simulink model "untitled1"  (R2022a)
settings: Solver=VariableStepAuto  StartTime=0.0  StopTime=2  MaxStep=0.005  RelTol=1e-3
values from neighbouring files (symbols this model uses):
  D_1 = 0.0001    [WS.m]
  D_2 = 0.0001    [WS.m]
  E_1 = 8.25 * 10^4    (= 82500)    [WS.m]
  E_2 = 8.25 * 10^4    (= 82500)    [WS.m]
  gy = 0    [WS.m]
  gz = 0    [WS.m]
  Imx_1 = 1.0053e-07    [WS.m]
  Imx_2 = 1.0053e-07    [WS.m]
  Ix_1 = 10^-5    (= 1e-05)    [WS.m]
  Ix_2 = 10^-5    (= 1e-05)    [WS.m]
  k_1_0 = 0.1    [WS.m]
  k_2_0 = 0.1    [WS.m]
  k_dot_1_0 = 0    [WS.m]
  k_dot_2_0 = 0    [WS.m]
  l_1 = 0.05    [WS.m]
  l_2 = 0.05    [WS.m]
  m_1 = 0.08    [WS.m]
  m_2 = 0.08    [WS.m]
  p_tendon_0 = [0.012,0,0]    [WS.m]
  p_tendon_1 = [0.012,0,0]    [WS.m]
  p_tendon_2 = [0.012,0,0]    [WS.m]
libraries: slpidlib x1, matrix_library x1
settings Model: Creator=luca  LastModifiedBy=atled
settings SolverCC: MaxConsecutiveMinStep=20

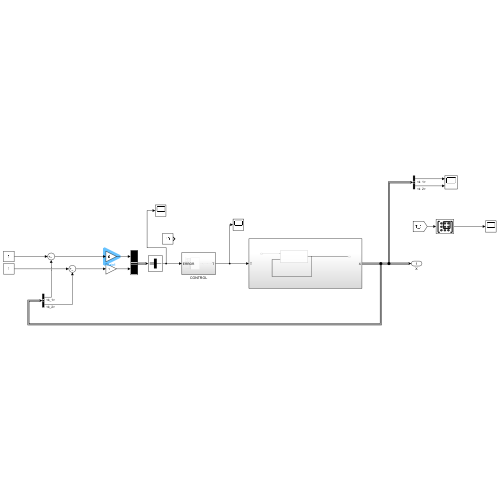
[thumbnail: Simulink's stored preview of the top-level diagram]
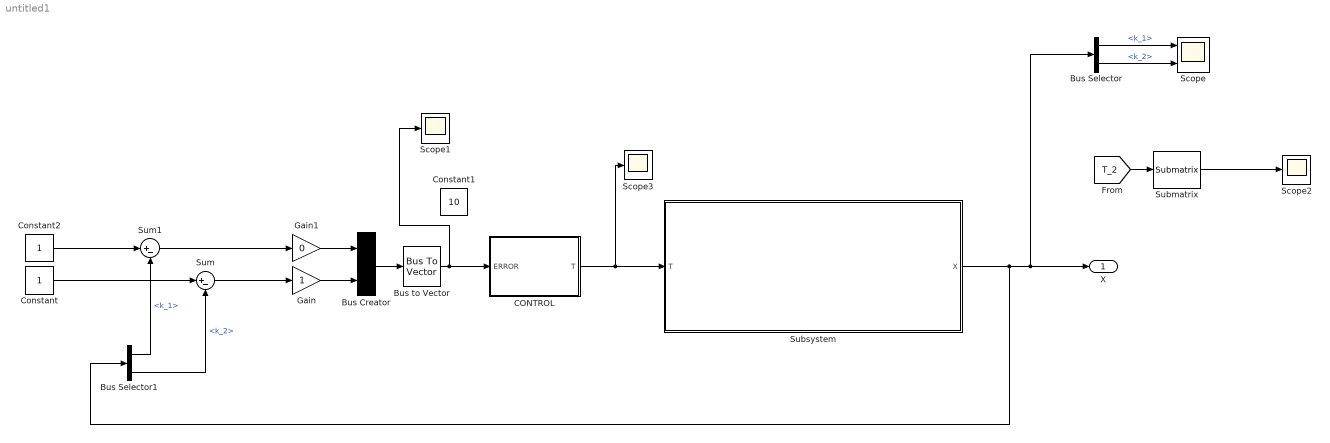
== system untitled1 ==
  Bus Creator : BusCreator  Inputs=2
  Bus Selector : BusSelector  OutputSignals=q.k_1,q.k_2
  Bus Selector1 : BusSelector  OutputSignals=q.k_1,q.k_2
  Bus to Vector : BusToVector
  CONTROL : Subsystem
  Constant : Constant  VectorParams1D=off
  Constant1 : Constant  Value=10  VectorParams1D=off
  Constant2 : Constant  VectorParams1D=off
  Gain : Gain
  Gain1 : Gain  Gain=0
  Scope : Scope  NumInputPorts=2
  Scope1 : Scope
  Scope2 : Scope
  Scope3 : Scope
  Submatrix : matrix_library/Submatrix  RowSpan=Range of rows  RowStartMode=Index  RowStartIndex=1  RowEndMode=Index  RowEndIndex=3  ColSpan=One column  ColStartMode=Last  ColStartIndex=1  ColEndMode=Last  ColEndIndex=1
      settings: SourceProductBaseCode=SL
  Subsystem : Subsystem
  Sum : Sum  Inputs=|+-
  Sum1 : Sum  Inputs=|+-
  X : Outport
  wires:
  Subsystem/1(X) -> Bus Selector1/1, Bus Selector/1, X/1
  Bus Selector/1 -> Scope/1  "<k_1>"
  Bus Selector/2 -> Scope/2  "<k_2>"
  Constant/1 -> Sum/1
  [T_2] -> Submatrix/1
  Submatrix/1 -> Scope2/1
  Sum/1 -> Gain/1
  Constant2/1 -> Sum1/1
  Bus Selector1/1 -> Sum1/2  "<k_1>"
  Bus Selector1/2 -> Sum/2  "<k_2>"
  Sum1/1 -> Gain1/1
  Bus to Vector/1 -> Scope1/1, CONTROL/1(ERROR)
  Gain1/1 -> Bus Creator/1
  Gain/1 -> Bus Creator/2
  CONTROL/1(T) -> Scope3/1, Subsystem/1(T)
  Bus Creator/1 -> Bus to Vector/1

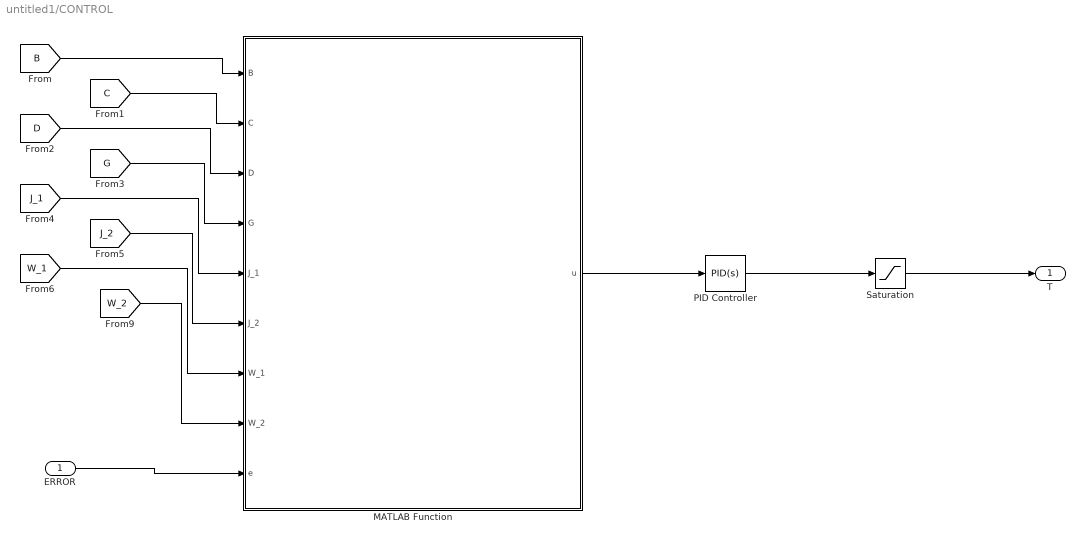
== system untitled1/CONTROL ==
  ERROR : Inport
  MATLAB Function : MATLAB Function  TreatAsAtomicUnit=on
  PID Controller : slpidlib/PID Controller  Controller=PID  Form=Parallel  TimeDomain=Continuous-time  UseExternalTs=off  SampleTime=-1  IntegratorMethod=Forward Euler  FilterMethod=Forward Euler  ControllerParametersSource=internal  P=-3  I=0  UseKiTs=off  D=0.02  N=100  UseFilter=on  TunerSelectOption=Transfer Function Based (PID Tuner App)  InitialConditionSource=internal  InitialConditionForIntegrator=0  InitialConditionForFilter=0  DifferentiatorICPrevScaledInput=0  ExternalReset=none  TrackingMode=off  Kt=1  LimitOutput=off  SatLimitsSource=internal  UpperSaturationLimit=inf  LowerSaturationLimit=-inf  LinearizeAsGain=on  AntiWindupMode=none  Kb=1  POutMin=[]  POutMax=[]  IOutMin=[]  IOutMax=[]  DOutMin=[]  DOutMax=[]  NOutMin=[]  NOutMax=[]  SumOutMin=[]  SumOutMax=[]  SaturationOutMin=[]  SaturationOutMax=[]  PParamMin=[]  PParamMax=[]  IParamMin=[]  IParamMax=[]  DParamMin=[]  DParamMax=[]  NParamMin=[]  NParamMax=[]  KbParamMin=[]  KbParamMax=[]  KtParamMin=[]  KtParamMax=[]  KbOutMin=[]  KbOutMax=[]  KtOutMin=[]  KtOutMax=[]  IntegratorOutMin=[]  IntegratorOutMax=[]  FilterOutMin=[]  FilterOutMax=[]  SumI1OutMin=[]  SumI1OutMax=[]  SumI2OutMin=[]  SumI2OutMax=[]  SumI3OutMin=[]  SumI3OutMax=[]  SumI4OutMin=[]  SumI4OutMax=[]  SumDOutMin=[]  SumDOutMax=[]  DifferentiatorOutMin=[]  DifferentiatorOutMax=[]  FilterDiffOutCoefMin=[]  FilterDiffOutCoefMax=[]  ReciprocalOutMin=[]  ReciprocalOutMax=[]  SumDenOutMin=[]  SumDenOutMax=[]  SumNumOutMin=[]  SumNumOutMax=[]  DivideOutMin=[]  DivideOutMax=[]  UdiffTsProdOutMin=[]  UdiffTsProdOutMax=[]  NTsProdOutMin=[]  NTsProdOutMax=[]  UintegralTsProdOutMin=[]  UintegralTsProdOutMax=[]  UngainTsProdOutMin=[]  UngainTsProdOutMax=[]  IntegratorContinuousStateAttributes=''  IntegratorStateMustResolveToSignalObject=off  IntegratorRTWStateStorageClass=Auto  FilterContinuousStateAttributes=''  FilterStateMustResolveToSignalObject=off  FilterRTWStateStorageClass=Auto  ParallelPVariant=InternalParameters  IdealPVariant=Disabled  IVariant=InternalParameters  DVariant=InternalParameters  IntegratorVariant=Continuous  SatVariant=Disabled  AWVariant=Passthrough  PCopyVariant=Disabled  TRVariant=Disabled  FdbkBlocksVariant=Forward  IdealPFdbkVariant=Disabled  SatFdbkVariant=Disabled  DerivativeFilterVariant=ContFilter  NVariant=InternalParameters  NCopyVariant=Disabled  FilterICVariant=InternalICsFilter  IntegratorICVariant=InternalICs  ExternalResetVariant=Disabled  TRSumVariant=Passthrough  SumFdbkVariant=Disabled  SumVariant=Sum_PID  TsampFilterVariant=InternalTs  TsampNgainVariant=Passthrough  TsampIntegralVariant=Passthrough  ExternalSaturationOutDataTypeStr=Inherit: Same as second input  aMode=0
  Saturation : Saturate  UpperLimit=50  LowerLimit=0
  T : Outport
  wires:
  [B] -> MATLAB Function/1(B)
  [C] -> MATLAB Function/2(C)
  [J_1] -> MATLAB Function/5(J_1)
  [G] -> MATLAB Function/4(G)
  [W_2] -> MATLAB Function/8(W_2)
  [J_2] -> MATLAB Function/6(J_2)
  [D] -> MATLAB Function/3(D)
  [W_1] -> MATLAB Function/7(W_1)
  ERROR/1 -> MATLAB Function/9(e)
  PID Controller/1 -> Saturation/1
  MATLAB Function/1(u) -> PID Controller/1
  Saturation/1 -> T/1

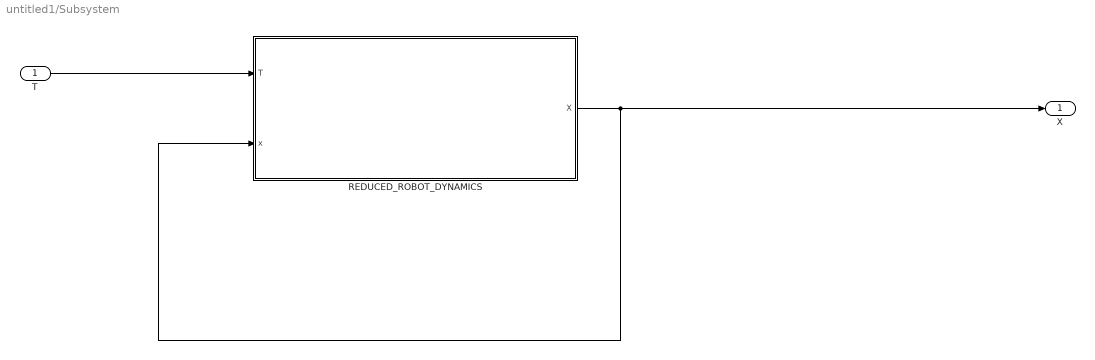
== system untitled1/Subsystem ==
  T : Inport
  REDUCED_ROBOT_DYNAMICS : Subsystem
  X : Outport
  wires:
  T/1 -> REDUCED_ROBOT_DYNAMICS/1(T)
  REDUCED_ROBOT_DYNAMICS/1(X) -> X/1, REDUCED_ROBOT_DYNAMICS/2(x)

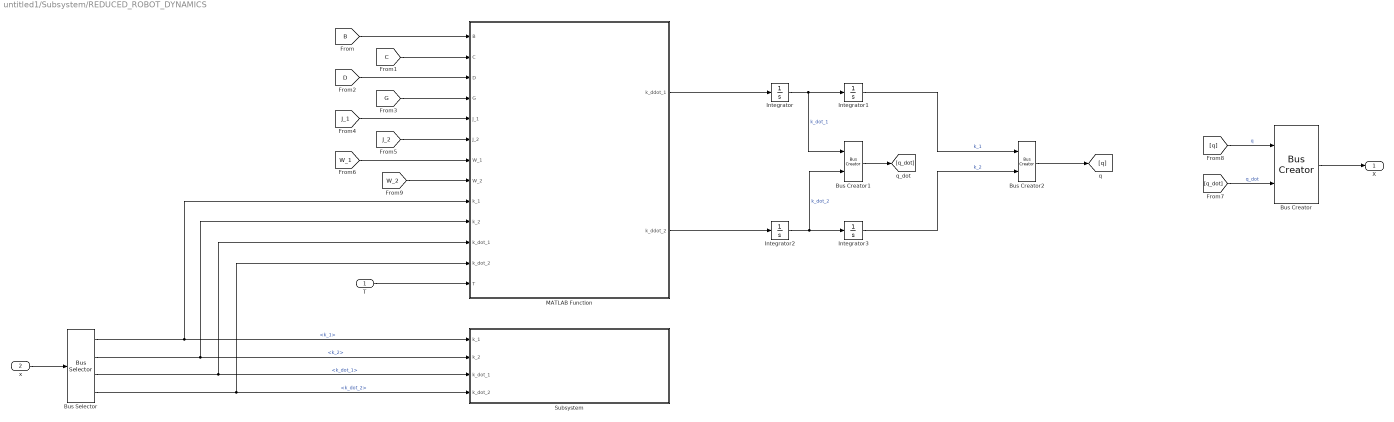
== system untitled1/Subsystem/REDUCED_ROBOT_DYNAMICS ==
  T : Inport
  x : Inport  Port=2
  Bus Creator : BusCreator  Inputs=2
  Bus Creator1 : BusCreator  Inputs=2
  Bus Creator2 : BusCreator  Inputs=2
  Bus Selector : BusSelector  OutputSignals=q.k_1,q.k_2,q_dot.k_dot_1,q_dot.k_dot_2
  Integrator : Integrator  InitialCondition=k_dot_1_0
  Integrator1 : Integrator  InitialCondition=k_1_0
  Integrator2 : Integrator  InitialCondition=k_dot_2_0
  Integrator3 : Integrator  InitialCondition=k_2_0
  MATLAB Function : MATLAB Function  TreatAsAtomicUnit=on
  Subsystem : Subsystem
  X : Outport
  wires:
  T/1 -> MATLAB Function/13(T)
  Bus Creator/1 -> X/1
  Bus Selector/1 -> MATLAB Function/9(k_1), Subsystem/1(k_1)  "<k_1>"
  Integrator2/1 -> Bus Creator1/2, Integrator3/1  "k_dot_2"
  [q] -> Bus Creator/1  "q"
  [q_dot] -> Bus Creator/2  "q_dot"
  [B] -> MATLAB Function/1(B)
  [W_1] -> MATLAB Function/7(W_1)
  [J_2] -> MATLAB Function/6(J_2)
  x/1 -> Bus Selector/1
  Integrator/1 -> Bus Creator1/1, Integrator1/1  "k_dot_1"
  [C] -> MATLAB Function/2(C)
  Bus Creator2/1 -> [q]
  Integrator3/1 -> Bus Creator2/2  "k_2"
  MATLAB Function/1(k_ddot_1) -> Integrator/1
  Bus Creator1/1 -> [q_dot]
  [D] -> MATLAB Function/3(D)
  MATLAB Function/2(k_ddot_2) -> Integrator2/1
  Bus Selector/4 -> MATLAB Function/12(k_dot_2), Subsystem/4(k_dot_2)  "<k_dot_2>"
  Bus Selector/3 -> MATLAB Function/11(k_dot_1), Subsystem/3(k_dot_1)  "<k_dot_1>"
  Integrator1/1 -> Bus Creator2/1  "k_1"
  [J_1] -> MATLAB Function/5(J_1)
  Bus Selector/2 -> MATLAB Function/10(k_2), Subsystem/2(k_2)  "<k_2>"
  [G] -> MATLAB Function/4(G)
  [W_2] -> MATLAB Function/8(W_2)

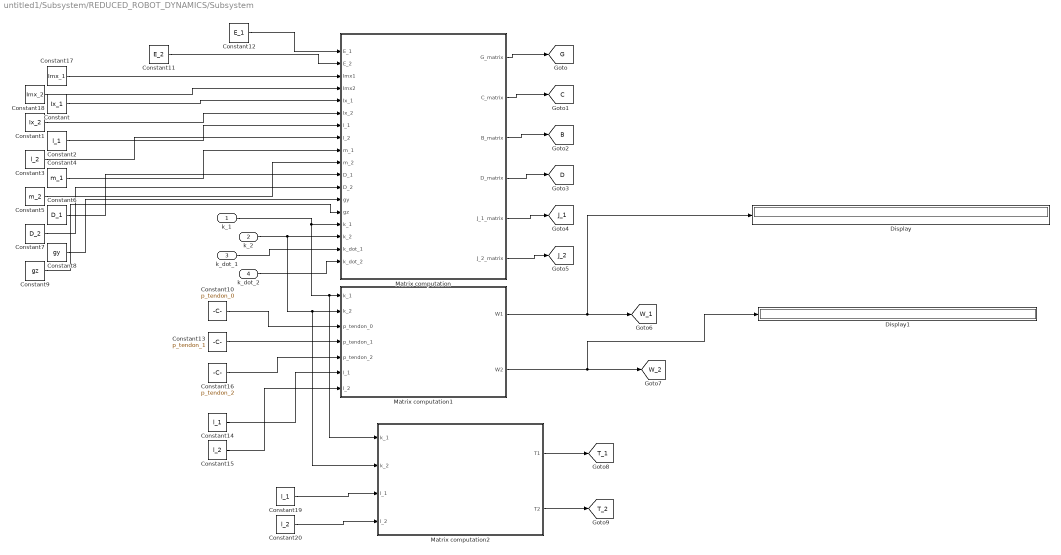
== system untitled1/Subsystem/REDUCED_ROBOT_DYNAMICS/Subsystem ==
  k_1 : Inport
  k_2 : Inport  Port=2
  k_dot_1 : Inport  Port=3
  k_dot_2 : Inport  Port=4
  Constant : Constant  Value=Ix_1
  Constant1 : Constant  Value=Ix_2
  Constant10 : Constant  Value=p_tendon_0
  Constant11 : Constant  Value=E_2
  Constant12 : Constant  Value=E_1
  Constant13 : Constant  Value=p_tendon_1
  Constant14 : Constant  Value=l_1
  Constant15 : Constant  Value=l_2
  Constant16 : Constant  Value=p_tendon_2
  Constant17 : Constant  Value=Imx_1
  Constant18 : Constant  Value=Imx_2
  Constant19 : Constant  Value=l_1
  Constant2 : Constant  Value=l_1
  Constant20 : Constant  Value=l_2
  Constant3 : Constant  Value=l_2
  Constant4 : Constant  Value=m_1
  Constant5 : Constant  Value=m_2
  Constant6 : Constant  Value=D_1
  Constant7 : Constant  Value=D_2
  Constant8 : Constant  Value=gy
  Constant9 : Constant  Value=gz
  Display : Display
  Display1 : Display
  Matrix computation : MATLAB Function  TreatAsAtomicUnit=on
  Matrix computation1 : MATLAB Function  TreatAsAtomicUnit=on
  Matrix computation2 : MATLAB Function  TreatAsAtomicUnit=on
  tag scope: B=global, C=global, D=global, G=global, J_1=global, J_2=global, T_1=global, T_2=global, W_1=global, W_2=global
  wires:
  k_2/1 -> Matrix computation2/2(k_2), Matrix computation1/2(k_2), Matrix computation/16(k_2)
  k_dot_1/1 -> Matrix computation/17(k_dot_1)
  Constant7/1 -> Matrix computation/12(D_2)
  Matrix computation/1(G_matrix) -> [G]
  Constant3/1 -> Matrix computation/8(l_2)
  Matrix computation/6(J_2_matrix) -> [J_2]
  k_dot_2/1 -> Matrix computation/18(k_dot_2)
  Constant6/1 -> Matrix computation/11(D_1)
  Matrix computation/3(B_matrix) -> [B]
  Constant2/1 -> Matrix computation/7(l_1)
  Constant5/1 -> Matrix computation/10(m_2)
  Constant4/1 -> Matrix computation/9(m_1)
  Matrix computation/4(D_matrix) -> [D]
  Matrix computation/2(C_matrix) -> [C]
  Constant1/1 -> Matrix computation/6(Ix_2)
  k_1/1 -> Matrix computation2/1(k_1), Matrix computation1/1(k_1), Matrix computation/15(k_1)
  Matrix computation/5(J_1_matrix) -> [J_1]
  Constant8/1 -> Matrix computation/13(gy)
  Constant/1 -> Matrix computation/5(Ix_1)
  Constant9/1 -> Matrix computation/14(gz)
  Constant15/1 -> Matrix computation1/7(l_2)
  Constant14/1 -> Matrix computation1/6(l_1)
  Constant16/1 -> Matrix computation1/5(p_tendon_2)
  Constant13/1 -> Matrix computation1/4(p_tendon_1)
  Matrix computation1/1(W1) -> Display/1, [W_1]
  Matrix computation1/2(W2) -> Display1/1, [W_2]
  Constant10/1 -> Matrix computation1/3(p_tendon_0)
  Constant12/1 -> Matrix computation/1(E_1)
  Constant11/1 -> Matrix computation/2(E_2)
  Constant17/1 -> Matrix computation/3(Imx1)
  Constant18/1 -> Matrix computation/4(Imx2)
  Constant20/1 -> Matrix computation2/4(l_2)
  Constant19/1 -> Matrix computation2/3(l_1)
  Matrix computation2/1(T1) -> [T_1]
  Matrix computation2/2(T2) -> [T_2]

== matlab function untitled1/Subsystem/REDUCED_ROBOT_DYNAMICS/Subsystem/Matrix computation2 ==
  data: k_1 input; k_2 input; T1 output; l_1 input; l_2 input; T2 output
function [T1,T2] = fcn(k_1,k_2,l_1,l_2)
T1 = g_1(k_1,l_1);
T2 = g_2(k_1/l_1,k_2/l_2,l_1,l_2);

== matlab function untitled1/Subsystem/REDUCED_ROBOT_DYNAMICS/Subsystem/Matrix computation ==
  data: E_1 input; E_2 input; Imx1 input; Imx2 input; Ix_1 input; G_matrix output; Ix_2 input; l_1 input; l_2 input; m_1 input; m_2 input; D_1 input; D_2 input; gy input; gz input; k_1 input; k_2 input; k_dot_1 input; k_dot_2 input; C_matrix output; B_matrix output; D_matrix output; J_1_matrix output; J_2_matrix output
function [G_matrix,C_matrix,B_matrix,D_matrix,J_1_matrix,J_2_matrix] = fcn(E_1,E_2,Imx1,Imx2,Ix_1, Ix_2 , l_1,l_2,m_1,m_2,D_1,D_2,gy,gz, k_1 , k_2 ,k_dot_1, k_dot_2)
G_matrix = G(E_1,E_2,Imx1,Imx2,gy,gz,k_1,k_2,l_1,l_2,m_1,m_2);
C_matrix = C(Ix_1,Ix_2,k_1,k_2,k_dot_1,k_dot_2,l_1,l_2,m_1,m_2);
B_matrix =  B(Ix_1,Ix_2,k_1,k_2,l_1,l_2,m_1,m_2);
D_matrix = diag([D_1,D_2]);
J_1_matrix = J_1(k_1,l_1);
J_2_matrix = J_2(k_1,k_2,l_1,l_2);

== matlab function untitled1/Subsystem/REDUCED_ROBOT_DYNAMICS/MATLAB Function ==
  data: B input; k_ddot_1 output size=1; C input; D input; G input; J_1 input; J_2 input; W_1 input; W_2 input; k_1 input; k_2 input; k_dot_1 input; k_dot_2 input; T input; k_ddot_2 output size=1
function [k_ddot_1,k_ddot_2] = fcn(B,C,D,G,J_1,J_2,W_1,W_2,k_1,k_2,k_dot_1,k_dot_2,T)

q = [k_1,k_2]';
q_dot = [k_dot_1,k_dot_2]';
A = [ J_1(1:6,1)' * W_1 ; J_2(1:6,2)' * W_2 ]
q_ddot = - B^-1 * (C * q_dot + D* q_dot + G - A * (-T) );
k_ddot_1 = q_ddot(1,1);
k_ddot_2 = q_ddot(2,1);

== matlab function untitled1/Subsystem/REDUCED_ROBOT_DYNAMICS/Subsystem/Matrix computation1 ==
  data: k_1 input; k_2 input; p_tendon_0 input; p_tendon_1 input; W1 output; p_tendon_2 input; l_1 input; l_2 input; W2 output
function [W1,W2] = fcn(k_1,k_2,p_tendon_0,p_tendon_1,p_tendon_2,l_1,l_2)
T_0 = eye(4);
T_1 = g_1(k_1\l_1,l_1);
T_2 = g_2(k_1\l_1,k_2\l_2,l_1,l_2);
O_0 = T_0(1:3,4);
O_1 = T_1(1:3,4);
O_2 = T_2(1:3,4);

P_1_0 = O_0 + p_tendon_0;
P_1_1 = O_1 + p_tendon_1;
P_1_2 = O_2 + p_tendon_2;

O0O1 = vectord(O_0,O_1);
O1O2 = vectord(O_1,O_2);

O0P0 = vectord(O_0,P_1_0);
O1P1 = vectord(O_1,P_1_1);
O2P2 = vectord(O_2,P_1_2);

P0P1 = vectord(P_1_0,P_1_1);
P1P2 = vectord(P_1_1,P_1_2);

W1 = zeros(6,1);
W2 = zeros(6,1);

F2 = P1P2 / norm(P1P2);

W2(1:3,1) = F2  ;
W2(4:6,1) = cross_form(O2P2) * F2 + cross_form( O1O2 ) * F2 ;


F2 = P1P2 / norm(P1P2);

W2(1:3,1) = F2  ;
W2(4:6,1) = cross_form(O2P2) * F2 + cross_form( O1O2 ) * F2 ;


F1 = - P0P1 / norm(P0P1) + P1P2 / norm(P1P2);
W1(1:3,1) = F1 + F2;
W1(4:6,1) = cross_form(O1P1) * (F1) + cross_form( O0O1 ) * F1 + W2(4:6,1);

== matlab function untitled1/CONTROL/MATLAB Function ==
  data: B input; u output; C input; D input; G input; J_1 input; J_2 input; W_1 input; W_2 input; e input
function u = fcn(B,C,D,G,J_1,J_2,W_1,W_2,e)
A = [ J_1(1:6,1)' * W_1 ; J_2(1:6,2)' * W_2 ];
u =  pinv(A) * e
